simulink model "Pendulo"  (R2021a)
settings: Solver=VariableStepAuto  StartTime=0.0  StopTime=10.0  RelTol=1e-3
values from neighbouring files (symbols this model uses):
  l = 1    [script.m]
  m = 2    [script.m]
  T2 = 10    [script.m]
  w0 = sqrt(g/l)    [script.m]
settings Model: Creator=taffarel55  LastModifiedBy=taffarel55

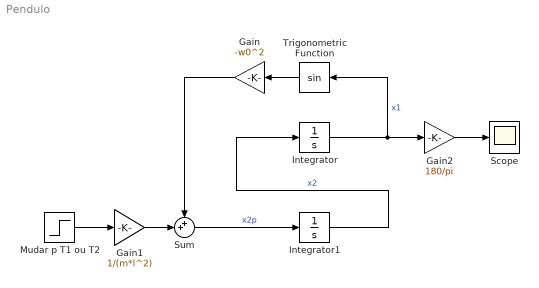
== system Pendulo ==
  Gain : Gain  Gain=-w0^2
  Gain1 : Gain  Gain=1/(m*l^2)
  Gain2 : Gain  Gain=180/pi
  Integrator : Integrator
  Integrator1 : Integrator
  Mudar p T1 ou T2 : Step  After=T2  SampleTime=0
  Scope : Scope
  Sum : Sum  Inputs=++|
  Trigonometric Function : Trigonometry
  wires:
  Integrator/1 -> Gain2/1, Trigonometric Function/1  "x1"
  Sum/1 -> Integrator1/1  "x2p"
  Integrator1/1 -> Integrator/1  "x2"
  Trigonometric Function/1 -> Gain/1
  Gain/1 -> Sum/1
  Gain1/1 -> Sum/2
  Mudar p T1 ou T2/1 -> Gain1/1
  Gain2/1 -> Scope/1
